simulink model "subsystem"  (Simulink 7.5)
settings: Solver=ode45  StartTime=0.0  StopTime=10.0  RelTol=1e-3
settings Model: Creator=lm  LastModifiedBy=lm

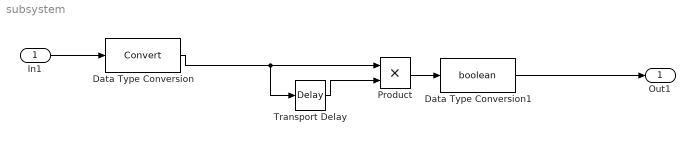
== system subsystem ==
  In1 : Inport  OutDataType=fixdt(1, 16)  OutScaling=2^0
  Data Type Conversion : DataTypeConversion  OutDataType=fixdt(1, 16)  OutScaling=2^0
  Data Type Conversion1 : DataTypeConversion  OutDataTypeMode=boolean  OutDataType=fixdt(1, 16)  OutScaling=2^0  OutDataTypeStr=boolean
  Product : Product  OutDataType=fixdt(1, 16)  OutScaling=2^0  RndMeth=Zero
  Transport Delay : TransportDelay
  Out1 : Outport  OutDataType=fixdt(1, 16)  OutScaling=2^0
  wires:
  Transport Delay/1 -> Product/2
  Data Type Conversion/1 -> Product/1, Transport Delay/1
  In1/1 -> Data Type Conversion/1
  Product/1 -> Data Type Conversion1/1
  Data Type Conversion1/1 -> Out1/1
